simulink subsystem "tehrani_tissue_compartment_v2"  (R2020b)
settings: Solver=VariableStepAuto  StartTime=0.0  StopTime=10.0  RelTol=1e-3
settings Model: Creator=RH  LastModifiedBy=fonck

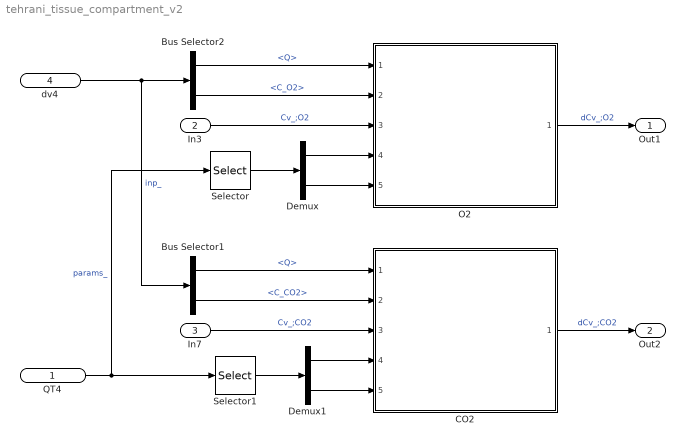
== system tehrani_tissue_compartment_v2 ==
  QT4 : Inport  PortDimensions=3
  In3 : Inport  Port=2  Unit=1
  In7 : Inport  Port=3  Unit=1
  dv4 : Inport  Port=4  OutDataTypeStr=Bus: BloodGasFlow
  Bus Selector1 : BusSelector  OutputSignals=Q,C_CO2
  Bus Selector2 : BusSelector  OutputSignals=Q,C_O2
  CO2 : Subsystem  ReferencedSubsystem=tehrani_tissue_mass_balance_v3
  Demux : Demux  Outputs=2
  Demux1 : Demux  Outputs=2
  O2 : Subsystem  ReferencedSubsystem=tehrani_tissue_mass_balance_v3
  Selector : Selector  InputPortWidth=3  IndexOptions=Index vector (dialog)  Indices=[2 1]  OutputSizes=1
  Selector1 : Selector  InputPortWidth=3  IndexOptions=Index vector (dialog)  Indices=[3 1]  OutputSizes=1
  Out1 : Outport  Unit=1/s
  Out2 : Outport  Port=2  Unit=1/s
  wires:
  Bus Selector2/2 -> O2/2  "<C_O2>"
  Bus Selector1/2 -> CO2/2  "<C_CO2>"
  CO2/1 -> Out2/1  "dCv_;CO2"
  O2/1 -> Out1/1  "dCv_;O2"
  In3/1 -> O2/3  "Cv_;O2"
  In7/1 -> CO2/3  "Cv_;CO2"
  dv4/1 -> Bus Selector2/1, Bus Selector1/1  "inp_"
  Bus Selector2/1 -> O2/1  "<Q>"
  Bus Selector1/1 -> CO2/1  "<Q>"
  QT4/1 -> Selector1/1, Selector/1  "params_"
  Demux/2 -> O2/5
  Demux/1 -> O2/4
  Selector/1 -> Demux/1
  Selector1/1 -> Demux1/1
  Demux1/1 -> CO2/4
  Demux1/2 -> CO2/5
